simulink model "experiment"  (R2016b)
settings: Solver=VariableStepAuto  StartTime=0.0  StopTime=15  MaxStep=0.05  RelTol=1e-3
model workspace (MAT data in the model file):
  GREEN_TIME = Simulink.Parameter
  GREEN_TIME.Value = 4
  GREEN_TIME.DataType = 'double'
  GREEN_TIME.Dimensions = [1 1]
  MIN_SAFE_DIST = Simulink.Parameter
  MIN_SAFE_DIST.Value = 1
  MIN_SAFE_DIST.DataType = 'double'
  MIN_SAFE_DIST.Dimensions = [1 1]
  PCROSS_TIME = Simulink.Parameter
  PCROSS_TIME.Value = 3
  PCROSS_TIME.DataType = 'double'
  PCROSS_TIME.Dimensions = [1 1]
  V_MIN = Simulink.Parameter
  V_MIN.Value = 0.25
  V_MIN.DataType = 'double'
  V_MIN.Dimensions = [1 1]
  V_TURN = Simulink.Parameter
  V_TURN.Value = 1.2
  V_TURN.DataType = 'double'
  V_TURN.Dimensions = [1 1]
  WORLD_SIZE = Simulink.Parameter
  WORLD_SIZE.Value = 8
  WORLD_SIZE.DataType = 'double'
  WORLD_SIZE.Dimensions = [1 1]
  YELLOW_TIME = Simulink.Parameter
  YELLOW_TIME.Value = 1
  YELLOW_TIME.DataType = 'double'
  YELLOW_TIME.Dimensions = [1 1]
  dt = Simulink.Parameter
  dt.Value = 0.05
  dt.DataType = 'double'
  dt.DocUnits = 'sec'
  dt.Dimensions = [1 1]
values from neighbouring files (symbols this model uses):
  D = ch.find('-isa','Stateflow.Data','-and','Name','D')    [createVehicle.m]    (also in initModelParams.m)
  MIN_SAFE_DIST = 1    [stateflowSim.m]
  V = ch.find('-isa','Stateflow.Data','-and','Name','V')    [createVehicle.m]    (also in initModelParams.m)
  WORLD_SIZE = 8    [offlineSim.m]    (also in stateflowSim.m)
  X = ch.find('-isa','Stateflow.Data','-and','Name','X')    [createVehicle.m]    (also in initModelParams.m)
undefined symbols (not defined in the file or in its folder): Stateflow
libraries: libraries x25
settings Model: Creator=larry  LastModifiedBy=larry
settings SolverCC: ZeroCrossControl=DisableAll  AutoInsertRateTranBlk=on

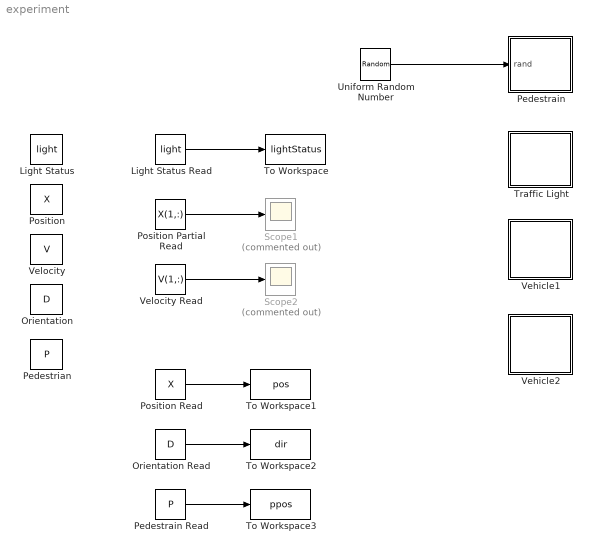
== system experiment ==
  Light Status : DataStoreMemory  DataStoreName=light  ShowAdditionalParam=off  OutDataTypeStr=double  Dimensions=1
  Light Status Read : DataStoreRead  DataStoreName=light
  Orientation : DataStoreMemory  DataStoreName=D  InitialValue=[1 1;0 0]  ShowAdditionalParam=off  OutDataTypeStr=double
  Orientation Read : DataStoreRead  DataStoreName=D
  Pedestrain : Stateflow chart  TreatAsAtomicUnit=on
  Pedestrain Read : DataStoreRead  DataStoreName=P
  Pedestrian : DataStoreMemory  DataStoreName=P  InitialValue=[-1; -1; -1; -1]  ShowAdditionalParam=off  OutDataTypeStr=double
  Position : DataStoreMemory  DataStoreName=X  InitialValue=[-5 -4;-0.5 -0.5]  ShowAdditionalParam=off  OutDataTypeStr=double
  Position Read : DataStoreRead  DataStoreName=X
  Position Partial Read : DataStoreRead  DataStoreName=X  DataStoreElements=X(1,:)
  Scope1 : Scope  Commented=on
  Scope2 : Scope  Commented=on
  To Workspace : ToWorkspace  VariableName=lightStatus  SampleTime=-1
  To Workspace1 : ToWorkspace  VariableName=pos  SampleTime=-1
  To Workspace2 : ToWorkspace  VariableName=dir  SampleTime=-1
  To Workspace3 : ToWorkspace  VariableName=ppos  SampleTime=-1
  Traffic Light : Stateflow chart  TreatAsAtomicUnit=on
  Uniform Random Number : UniformRandomNumber  Minimum=0  Maximum=5  SampleTime=0.05
  Vehicle1 : Stateflow chart  TreatAsAtomicUnit=on
  Vehicle2 : Stateflow chart  TreatAsAtomicUnit=on
  Velocity : DataStoreMemory  DataStoreName=V  InitialValue=[0 0;0 0]  ShowAdditionalParam=off  OutDataTypeStr=double
  Velocity Read : DataStoreRead  DataStoreName=V  DataStoreElements=V(1,:)
  wires:
  Light Status Read/1 -> To Workspace/1
  Position Partial Read/1 -> Scope1/1
  Velocity Read/1 -> Scope2/1
  Position Read/1 -> To Workspace1/1
  Orientation Read/1 -> To Workspace2/1
  Uniform Random Number/1 -> Pedestrain/1(rand)
  Pedestrain Read/1 -> To Workspace3/1

== stateflow chart experiment/Vehicle1 ==
  note: Decision
  note: Perception
  note: Helper
  state GoStraight
    state FreeDriving
    state Follow
      en:
      front = frontCarIndex(this);
      state FollowBehind
    (default) -> GoStraight.FreeDriving [order 2]
    GoStraight.FreeDriving -> GoStraight.Follow : [hasFrontCar(this)]
    GoStraight.Follow -> GoStraight.FreeDriving : [frontCarHasLeft(this)]
    (default) -> GoStraight.Follow [order 1] : [hasFrontCar(this)]
  state Turn
    en:
    completed = false;
    state Right
      en:
      [pf,df] = ...
      prepareRight(this);
      ex:
      inter = resumeFromRight(this, df);
      state Turn
      state TurnStop
      (default) -> Turn.Right.Turn
      Turn.Right.TurnStop -> Turn.Right.Turn : [~hasPedestrian(this)]
      Turn.Right.Turn -> Turn.Right.TurnStop : [hasPedestrian(this)]
    state Left
      en:
      [pf, df] = ...
      prepareLeft(this);
      ex:
      inter = resumeFromLeft(this, df);
      state Turn
      state TurnStop
      (default) -> Turn.Left.Turn
      Turn.Left.TurnStop -> Turn.Left.Turn : [~hasPedestrian(this)]
      Turn.Left.Turn -> Turn.Left.TurnStop : [hasPedestrian(this)]
    (default) -> Right [order 1] : [decision == Decision.Right]
    (default) -> Left [order 2]
  state RoadIntersection
    state Normal
      state FreeDriving
        state AccToHighestRate
        state SlowDownToStop
        state SlowAdjust
        state RushToPass
        (default) -> (junction 88) [order 2]
        (default) -> AccToHighestRate [order 1] : [isGreen(this)]
        AccToHighestRate -> (junction 88) : [isYellow(this)]
        (junction 88) -> (junction 177) [order 2]
        (junction 88) -> RoadIntersection.Normal.FreeDriving.SlowAdjust [order 1] : [isStopped(this)]...
            | {obj = inter;}
        RoadIntersection.Normal.FreeDriving.SlowAdjust -> AccToHighestRate : [isGreen(this)]
        SlowDownToStop -> AccToHighestRate : [isGreen(this)]
        (junction 177) -> SlowDownToStop [order 1] : [isStoppable(this,inter)]...
            | {a_norm = requiredBrake(...
            | this,inter);}
        (junction 177) -> RushToPass [order 2]
      state Follow
        en:
        front = frontCarIndex(this);
        obj = X(:,front);
        du:
        obj = closestObj(this, obj, inter);
        state FollowBehind
        state NonStopFollow
        state SlowAdjust
        (default) -> (junction 164) [order 2]
        (default) -> RoadIntersection.Normal.Follow.FollowBehind [order 1] : [isGreen(this)]
        RoadIntersection.Normal.Follow.FollowBehind -> (junction 164) : [isYellow(this)]
        (junction 164) -> RoadIntersection.Normal.Follow.SlowAdjust [order 1] : [isStoppable(this,obj)]
        (junction 164) -> NonStopFollow [order 2]
        RoadIntersection.Normal.Follow.SlowAdjust -> RoadIntersection.Normal.Follow.FollowBehind : [isGreen(this)]
      (default) -> RoadIntersection.Normal.FreeDriving [order 2]
      (default) -> RoadIntersection.Normal.Follow [order 1] : [hasFrontCar(this)]
      RoadIntersection.Normal.FreeDriving -> RoadIntersection.Normal.Follow : [hasFrontCar(this)]
      RoadIntersection.Normal.Follow -> RoadIntersection.Normal.FreeDriving : [frontCarHasLeft(this)]
    state Pedestrian
      state EmergenceStop
    (default) -> Normal [order 2]
    Normal -> Pedestrian : [hasPedestrian(this)]
    Pedestrian -> Normal : [~hasPedestrian(this)]
    (default) -> Pedestrian [order 1] : [hasPedestrian(this)]
  (default) -> GoStraight
  Turn -> GoStraight : [completed]
  (junction 195) -> Turn [order 2]
  (junction 195) -> GoStraight [order 1] : [decision == Decision.Straight]
  RoadIntersection -> (junction 195) : [passStopLine(this)]
  GoStraight -> RoadIntersection : [isCloseTo(this,inter)]
  data: v_target function_input; a_norm function_input; this function_input; a_max function_input; this function_input; front function_input; this function_input; completed function_output; d2 function_input; p2 function_input; this function_input; p2 function_input; this function_input; completed function_output; d2 function_input; p2 function_input; this function_input; p2 function_input; self function_input; res function_output; self function_input; obj1 function_input; res function_output; obj2 function_input; self function_input; pos function_input; res function_output; self function_input; res function_output; self function_input; idx function_output; self function_input uint8 size=1; d function_input; newInnter function_output; self function_input; res function_output; pos function_input; self function_input; pos function_input; res function_output; self function_input uint8 size=1; d function_input; newInter function_output; self function_input; res function_output; self function_input uint8 size=1; p function_output; d function_output; self function_input uint8 size=1; p function_output; d function_output; self function_input; res function_output; self function_input; res function_output; self function_input; res function_output; v_target function_input; a_norm function_input; this function_input; a_norm function_input; this function_input; this function_input; a_norm function_input; obj function_input; v_target function_input; a_norm function_input; this function_input; a_max function_input; this function_input; front function_input; a_max function_input; this function_input; front function_input; this function_input; a_norm function_input; obj function_input; a_norm function_input; this function_input; self function_input uint8 size=1; res function_output boolean size=1; dt parameter double size=1 =0.05; this local uint8 =uint8(1); V data_store_memory; X data_store_memory size=[1 2]; D data_store_memory; A_MAX local double =2.5; V_MAX local double =2.5; light data_store_memory; inter local double size=[2 1] =[-1; -0.5]; MIN_SAFE_DIST parameter; a_norm local double size=1 =0; WORLD_SIZE parameter; front local uint8 size=1; obj local double size=[2 1]; V_MIN parameter; decision local Enum: Decision size=1 =Decision.Right; completed local boolean size=1 =false; P data_store_memory; df local double size=[2 1]; pf local double size=[2 1]
  function res = hasPedestrian(self):
    | function res = hasPedestrian(self)
    | 
    | if ~any(P ~= -1)
    |     res = false;
    |     return;
    | end
    | 
    | FARAWAY = 100;
    | 
    | pi = [-1 1 1 -1; -1 -1 1 1];
    | dp = [2 0 -2 0; 0 2 0 -2];
    | 
    | dx_norm = ones(4, 1) * FARAWAY;
    | x = X(:,self);
    | d = D(:,self);
    | 
    | for k=1:length(P)
    |     if P(k) ~= -1
    |         p = pi(:,k) + dp(:,k) * P(k); 
    |         dx = p - x;
    |         check = dot(dx, d);
    |         if check > 0
    |             dx_norm(k) = norm(dx);
    |             theta = acos(check/dx_norm(k));
    |             if rad2deg(theta) > 10
    |                 dx_norm(k) = FARAWAY;
    |             end
    |         end
    |     end
    | end
    | 
    | res = any(dx_norm <= 1 * MIN_SAFE_DIST);
  function res = closestObj(self, obj1, obj2):
    | function res = closestObj(self, obj1, obj2)
    | 
    | if isequal(obj1, obj2)
    |     res = obj1;
    |     return;
    | end
    | 
    | RANGE = 2*WORLD_SIZE;
    | 
    | x = X(:,self);
    | d = D(:,self);
    | 
    | dX = zeros(2, 1);
    | dX(1) = mod(dot(obj1 - x, d) + RANGE, RANGE);
    | dX(2) = mod(dot(obj2 - x, d) + RANGE, RANGE);
    | 
    | [~, index] = min(dX);
    | if index == 1
    |     res = obj1;
    | else
    |     res = obj2;
    | end
  function res = isStoppable(self,pos):
    | function res = isStoppable(self,pos)
    | 
    | x = X(:,self);
    | v = V(:,self);
    | d = D(:,self);
    | 
    | range = 2 * WORLD_SIZE;
    | diff = mod((dot(pos - x, d)+range), range) ;
    | dist = diff - MIN_SAFE_DIST;
    | 
    | v_norm = norm(v);
    | brake_dist = v_norm*v_norm/2.0/A_MAX;
    | res = (brake_dist <= dist);
  function res = passStopLine(self):
    | function res = passStopLine(self)
    | 
    | x = X(:,self);
    | d = D(:,self);
    | 
    | dx_norm = dot(inter - x, d);
    | res = (dx_norm <= 0);
  function idx = frontCarIndex(self):
    | function idx = frontCarIndex(self)
    | 
    | FARAWAY = 100;
    | RANGE = 2*WORLD_SIZE;
    | 
    | dx = zeros(size(X, 2), 1);
    | x = X(:,self);
    | v = V(:,self);
    | d = D(:,self);
    | 
    | for k=1:length(dx)
    |     dx(k) = dot(X(:,k) - x, d);
    |     dx(k) = mod((dx(k)+RANGE), RANGE);
    | end
    | 
    | % set zero dX to a large enough value
    | dx(dx == 0) = FARAWAY;
    | [~, idx] = min(dx);
    | idx = uint8(idx);
  function newInnter = resumeFromRight(self, d):
    | function newInnter = resumeFromRight(self, d)
    | 
    | x = X(:,self);
    | 
    | if isequal(d, [0; -1])
    |     x = [-0.5; -1];
    |     newInnter = [-0.5; 1];
    | elseif isequal(d, [0; 1])
    |     x = [0.5; 1];
    |     newInnter = [-0.5; -1];
    | elseif isequal(d, [1; 0])
    |     x = [1; -0.5];
    |     newInnter = [-1; -0.5];
    | elseif isequal(d, [-1; 0])
    |     x = [-1; 0.5];
    |     newInnter = [1; 0.5];
    | else
    |     error('Unknown orientation');
    | end
    | 
    | v = V(:,self);
    | 
    | X(:,self) = x;
    | V(:,self) = d * norm(v);
    | D(:,self) = d;
  function res = isCloseTo(self,pos):
    | function res = isCloseTo(self,pos)
    | 
    | x = X(:,self);
    | d = D(:,self);
    | 
    | dist = dot(pos-x, d);
    | res = ((dist > 0) && (dist <= 2.5*MIN_SAFE_DIST));
  function res = requiredBrake(self,pos):
    | function res = requiredBrake(self,pos)
    | 
    | x = X(:,self);
    | v = V(:,self);
    | d = D(:,self);
    | 
    | % add safe distance
    | range = 2 * WORLD_SIZE;
    | diff = mod((dot(pos - x, d)+range),range);
    | dist = diff - MIN_SAFE_DIST;
    | assert(dist >= 0);
    | 
    | vnorm = norm(v);
    | res = vnorm*vnorm/2/dist;
  function newInter = resumeFromLeft(self, d):
    | function newInter = resumeFromLeft(self, d)
    | 
    | x = X(:,self);
    | v = V(:,self);
    | 
    | if isequal(d, [1; 0])
    |     x = [1; -0.5];
    |     newInter = [-1; -0.5];
    | elseif isequal(d, [-1; 0])
    |     x = [-1; 0.5];
    |     newInter = [1; 0.5];
    | elseif isequal(d, [0; 1])
    |     x = [0.5; 1];
    |     newInter = [0.5; -1];
    | elseif isequal(d, [0; -1])
    |     x = [-0.5; -1];
    |     newInter = [-0.5; 1];
    | else
    |     error('Unknown orientation');
    | end
    | 
    | X(:,self) = x;
    | V(:,self) = d * norm(v);
    | D(:,self) = d;
  function res = isGreen(self):
    | function res = isGreen(self)
    | 
    | d = D(:,self);
    | 
    | % compute the corresponding traffic light
    | horizon = (abs(d(1)) ~= 0);
    | vertical = (abs(d(2)) ~= 0);
    | 
    | res = false;
    | if uint8(light) == 3 && horizon
    |     % horizontal: green, vertical: red
    |     res = true;
    | elseif uint8(light) == 1 && vertical
    |     % horizontal: red, vertical: green
    |     res = true;
    | end
  function [p, d] = prepareRight(self):
    | function [p, d] = prepareRight(self)
    | 
    | d0 = D(:,self);
    | p = [0; 0];
    | d = [0; 0];
    | 
    | if isequal(d0, [1; 0])
    |     p = [-0.5; -1];
    |     d = [0; -1];
    | elseif isequal(d0, [-1; 0])
    |     p = [0.5; 1];
    |     d = [0; 1];
    | elseif isequal(d0, [0; 1])
    |     p = [1; -0.5];
    |     d = [1; 0];
    | elseif isequal(d0, [0; -1])
    |     p = [-1; 0.5];
    |     d = [-1; 0];
    | else
    |     error('Unknown orientation');
    | end
  function [p, d] = prepareLeft(self):
    | function [p, d] = prepareLeft(self)
    | 
    | d0 = D(:,self);
    | p = [0; 0];
    | d = [0; 0];
    | 
    | if isequal(d0, [1; 0])
    |     p = [0.5; 1];
    |     d = [0; 1];
    | elseif isequal(d0, [-1; 0])
    |     p = [-0.5; -1];
    |     d = [0; -1];
    | elseif isequal(d0, [0; 1])
    |     p = [-1; 0.5];
    |     d = [-1; 0];
    | elseif isequal(d0, [0; -1])
    |     p = [1; -0.5];
    |     d = [1; 0];
    | else
    |     error('Unknown orientation');
    | end
  function res = isYellow(self):
    | function res = isYellow(self)
    | 
    | d = D(:,self);
    | 
    | % compute the corresponding traffic light
    | horizon = (abs(d(1)) ~= 0);
    | vertical = (abs(d(2)) ~= 0);
    | 
    | res = false;
    | if uint8(light) == 4 && horizon
    |     % horizontal: yellow, vertical: red
    |     res = true;
    | elseif uint8(light) == 2 && vertical
    |     % horizontal: red, vertical: yellow
    |     res = true;
    | end
  function res = hasFrontCar(self):
    | function res = hasFrontCar(self)
    | 
    | % constants
    | THRES = 2 * MIN_SAFE_DIST;
    | FARAWAY = 100;
    | RANGE = 2 * WORLD_SIZE;
    | 
    | res = false;
    | 
    | % row of X: coordinate, col of X: num of cars
    | num = size(X, 2);
    | if num == 1
    |     return;
    | end
    | 
    | dx = zeros(num, 1);
    | x = X(:,self);
    | d = D(:,self);
    | car_size = [0.3; 0.4];
    | 
    | for k=1:length(dx)
    |     
    |     % compute difference
    |     xdelta = X(:,k) - x;
    |     
    |     % parallel and vertical distance
    |     delta_p = dot(xdelta, d);
    |     delta_v = norm(xdelta - (d * delta_p));
    |     
    |     % vertical distance is larger than car width
    |     if delta_v < car_size(1)
    |         dx(k) = delta_p;
    |     else
    |         dx(k) = FARAWAY;
    |     end
    |     
    |     % a rounded world
    |     dx(k) = mod((dx(k)+RANGE), RANGE);
    | end
    | 
    | % set zero dX to a large enough value
    | dx(dx == 0) = FARAWAY;
    | closest = min(dx);
    | res = closest <= THRES;
  function res = frontCarHasLeft(self):
    | function res = frontCarHasLeft(self)
    | 
    | % Constants 
    | THRES = 2.5 * MIN_SAFE_DIST;
    | FARAWAY = 100;
    | RANGE = 2 * WORLD_SIZE;
    | 
    | % if only one car in the environment return directly
    | res = true;
    | num = size(X, 1);
    | if num == 1
    |     return;
    | end
    | 
    | % get the closet car index and its distance
    | dx = zeros(num, 1);
    | x = X(:,self);
    | d = D(:,self);
    | car_size = [0.3; 0.4];
    | 
    | for k=1:length(dx)
    |     
    |     xdelta = X(:,k) - x;
    |     xdelta_p = dot(xdelta, d);                  % parallel component
    |     xdelta_v = norm(xdelta - (d * xdelta_p));   % vertical component
    |     
    |     % when the vertical component is larger than the car width
    |     if xdelta_v < car_size(1)
    |         dx(k) = xdelta_p;
    |     else
    |         dx(k) = FARAWAY;
    |     end
    |     
    |     % since we are in the round world, normalize the distance if the 
    |     % front car is behind us 
    |     % a rounded world
    |     dx(k) = mod((dx(k)+RANGE), RANGE);
    | end
    | 
    | % set the zero dx to a large enough value for convenience
    | dx(dx == 0) = FARAWAY;
    | closest = min(dx);
    | res = closest > THRES;
  function res = isStopped(self):
    | function res = isStopped(self)
    | 
    | v = V(:,self);
    | d = D(:,self);
    | res = (dot(v, d) <= 0)||(norm(v) < V_MIN);

== stateflow chart experiment/Vehicle2 ==
  state Turn
    en:
    theta_in = 0;
    completed = false;
    state TurnLeft
    state TurnRight
    (default) -> TurnLeft [order 2]
    (default) -> TurnRight [order 1] : [decision == Decision.Right]
  state GoStraight
    state FreeDriving
    state Follow
      en:
      front = frontCarIndex(this);
      state FollowBehind
    (default) -> GoStraight.FreeDriving [order 2]
    GoStraight.FreeDriving -> GoStraight.Follow : [hasFrontCar(this)]
    GoStraight.Follow -> GoStraight.FreeDriving : [frontCarHasLeft(this)]
    (default) -> GoStraight.Follow [order 1] : [hasFrontCar(this)]
  state RoadIntersection
    state FreeDriving
      state AccToHighestRate
      state SlowDownToStop
      state SlowAdjust
      state RushToPass
      (default) -> (junction 88) [order 2]
      (default) -> AccToHighestRate [order 1] : [isGreen(this)]
      AccToHighestRate -> (junction 88) : [isYellow(this)]
      (junction 88) -> (junction 177) [order 2]
      (junction 88) -> RoadIntersection.FreeDriving.SlowAdjust [order 1] : [isStopped(this)]...
          | {obj = inter;}
      RoadIntersection.FreeDriving.SlowAdjust -> AccToHighestRate : [isGreen(this)]
      SlowDownToStop -> AccToHighestRate : [isGreen(this)]
      (junction 177) -> SlowDownToStop [order 1] : [isStoppable(this,inter)]...
          | {a_norm = requiredBrake(...
          | this,inter);}
      (junction 177) -> RushToPass [order 2]
    state Follow
      en:
      front = frontCarIndex(this);
      obj = X(:,front);
      du:
      obj = closestObj(this, obj, inter);
      state FollowBehind
      state NonStopFollow
      state SlowAdjust
      (default) -> (junction 164) [order 2]
      (default) -> RoadIntersection.Follow.FollowBehind [order 1] : [isGreen(this)]
      RoadIntersection.Follow.FollowBehind -> (junction 164) : [isYellow(this)]
      (junction 164) -> RoadIntersection.Follow.SlowAdjust [order 1] : [isStoppable(this,obj)]
      (junction 164) -> NonStopFollow [order 2]
      RoadIntersection.Follow.SlowAdjust -> RoadIntersection.Follow.FollowBehind : [isGreen(this)]
    (default) -> RoadIntersection.FreeDriving [order 2]
    (default) -> RoadIntersection.Follow [order 1] : [hasFrontCar(this)]
    RoadIntersection.FreeDriving -> RoadIntersection.Follow : [hasFrontCar(this)]
    RoadIntersection.Follow -> RoadIntersection.FreeDriving : [frontCarHasLeft(this)]
  (default) -> GoStraight
  Turn -> GoStraight : [completed]
  (junction 195) -> Turn [order 2]
  (junction 195) -> GoStraight [order 1] : [decision == Decision.Straight]
  RoadIntersection -> (junction 195) : [passStopLine(this)]
  GoStraight -> RoadIntersection : [isCloseTo(this,inter)]
  data: newInter function_output; this function_input; completed function_output; newInter function_output; this function_input; completed function_output; theta_in function_input; theta function_output; v_target function_input; a_norm function_input; this function_input; a_max function_input; this function_input; front function_input; self function_input; res function_output; self function_input; res function_output; self function_input; res function_output; pos function_input; self function_input; res function_output; self function_input; res function_output; self function_input; res function_output; self function_input; res function_output; v_target function_input; a_norm function_input; this function_input; a_norm function_input; this function_input; this function_input; a_norm function_input; obj function_input; v_target function_input; a_norm function_input; this function_input; a_max function_input; this function_input; front function_input; a_max function_input; this function_input; front function_input; this function_input; a_norm function_input; obj function_input; self function_input; obj1 function_input; res function_output; obj2 function_input; self function_input; idx function_output; self function_input; pos function_input; res function_output; self function_input; pos function_input; res function_output; self function_input uint8 size=1; res function_output boolean size=1; dt parameter double size=1 =0.05; this local uint8 =uint8(2); V data_store_memory; X data_store_memory size=[1 2]; D data_store_memory; A_MAX local double =2.5; V_MAX local double =2.5; light data_store_memory; inter local double size=[2 1] =[-1; -0.5]; MIN_SAFE_DIST parameter; a_norm local double size=1 =0; WORLD_SIZE parameter; front local uint8 size=1; obj local double size=[2 1]; V_MIN parameter; decision local Enum: Decision size=1 =Decision.Straight; completed local boolean size=1 =false; theta_in local double size=1 =0; theta_out local double size=1 =0
  function res = hasPedestrian(self):
    | function res = hasPedestrian(self)
    | 
    | FARAWAY = 100;
    | 
    | pi = [-1 1 1 -1; -1 -1 1 1];
    | dp = [2 0 -2 0; 0 2 0 -2];
    | 
    | dx_norm = ones(4, 1) * FARAWAY;
    | x = X(:,self);
    | d = D(:,self);
    | 
    | for k=1:length(P)
    |     if P(k) ~= -1
    |         p = pi(:,k) + dp * P(k); 
    |         dx = p - x;
    |         if dot(dx, d) > 0
    |             dx_norm(k) = norm(dx);
    |         end
    |     end
    | end
    | res = ~isempty(dx <= MIN_SAFE_DIST);
  function res = passStopLine(self):
    | function res = passStopLine(self)
    | 
    | x = X(:,self);
    | d = D(:,self);
    | 
    | dx_norm = dot(inter - x, d);
    | res = (dx_norm <= 0);
  function res = isCloseTo(self,pos):
    | function res = isCloseTo(self,pos)
    | 
    | x = X(:,self);
    | d = D(:,self);
    | 
    | dist = dot(pos-x, d);
    | res = ((dist > 0) && (dist <= 2.5*MIN_SAFE_DIST));
  function res = isGreen(self):
    | function res = isGreen(self)
    | 
    | d = D(:,self);
    | 
    | % compute the corresponding traffic light
    | horizon = (abs(d(1)) ~= 0);
    | vertical = (abs(d(2)) ~= 0);
    | 
    | res = false;
    | if uint8(light) == 3 && horizon
    |     % horizontal: green, vertical: red
    |     res = true;
    | elseif uint8(light) == 1 && vertical
    |     % horizontal: red, vertical: green
    |     res = true;
    | end
  function res = isYellow(self):
    | function res = isYellow(self)
    | 
    | d = D(:,self);
    | 
    | % compute the corresponding traffic light
    | horizon = (abs(d(1)) ~= 0);
    | vertical = (abs(d(2)) ~= 0);
    | 
    | res = false;
    | if uint8(light) == 4 && horizon
    |     % horizontal: yellow, vertical: red
    |     res = true;
    | elseif uint8(light) == 2 && vertical
    |     % horizontal: red, vertical: yellow
    |     res = true;
    | end
  function res = hasFrontCar(self):
    | function res = hasFrontCar(self)
    | 
    | % constants
    | THRES = 2 * MIN_SAFE_DIST;
    | FARAWAY = 100;
    | RANGE = 2 * WORLD_SIZE;
    | 
    | res = false;
    | 
    | % row of X: coordinate, col of X: num of cars
    | num = size(X, 2);
    | if num == 1
    |     return;
    | end
    | 
    | dx = zeros(num, 1);
    | x = X(:,self);
    | d = D(:,self);
    | car_size = [0.3; 0.4];
    | 
    | for k=1:length(dx)
    |     
    |     % compute difference
    |     xdelta = X(:,k) - x;
    |     
    |     % parallel and vertical distance
    |     delta_p = dot(xdelta, d);
    |     delta_v = norm(xdelta - (d * delta_p));
    |     
    |     % vertical distance is larger than car width
    |     if delta_v < car_size(1)
    |         dx(k) = delta_p;
    |     else
    |         dx(k) = FARAWAY;
    |     end
    |     
    |     % a rounded world
    |     dx(k) = mod((dx(k)+RANGE), RANGE);
    | end
    | 
    | % set zero dX to a large enough value
    | dx(dx == 0) = FARAWAY;
    | closest = min(dx);
    | res = closest <= THRES;
  function res = frontCarHasLeft(self):
    | function res = frontCarHasLeft(self)
    | 
    | % Constants 
    | THRES = 2.5 * MIN_SAFE_DIST;
    | FARAWAY = 100;
    | RANGE = 2 * WORLD_SIZE;
    | 
    | % if only one car in the environment return directly
    | res = true;
    | num = size(X, 1);
    | if num == 1
    |     return;
    | end
    | 
    | % get the closet car index and its distance
    | dx = zeros(num, 1);
    | x = X(:,self);
    | d = D(:,self);
    | car_size = [0.3; 0.4];
    | 
    | for k=1:length(dx)
    |     
    |     xdelta = X(:,k) - x;
    |     xdelta_p = dot(xdelta, d);                  % parallel component
    |     xdelta_v = norm(xdelta - (d * xdelta_p));   % vertical component
    |     
    |     % when the vertical component is larger than the car width
    |     if xdelta_v < car_size(1)
    |         dx(k) = xdelta_p;
    |     else
    |         dx(k) = FARAWAY;
    |     end
    |     
    |     % since we are in the round world, normalize the distance if the 
    |     % front car is behind us 
    |     % a rounded world
    |     dx(k) = mod((dx(k)+RANGE), RANGE);
    | end
    | 
    | % set the zero dx to a large enough value for convenience
    | dx(dx == 0) = FARAWAY;
    | closest = min(dx);
    | res = closest > THRES;
  function res = closestObj(self, obj1, obj2):
    | function res = closestObj(self, obj1, obj2)
    | 
    | if isequal(obj1, obj2)
    |     res = obj1;
    |     return;
    | end
    | 
    | RANGE = 2*WORLD_SIZE;
    | 
    | x = X(:,self);
    | d = D(:,self);
    | 
    | dX = zeros(2, 1);
    | dX(1) = mod(dot(obj1 - x, d) + RANGE, RANGE);
    | dX(2) = mod(dot(obj2 - x, d) + RANGE, RANGE);
    | 
    | [~, index] = min(dX);
    | if index == 1
    |     res = obj1;
    | else
    |     res = obj2;
    | end
  function idx = frontCarIndex(self):
    | function idx = frontCarIndex(self)
    | 
    | FARAWAY = 100;
    | RANGE = 2*WORLD_SIZE;
    | 
    | dx = zeros(size(X, 2), 1);
    | x = X(:,self);
    | v = V(:,self);
    | d = D(:,self);
    | 
    | for k=1:length(dx)
    |     dx(k) = dot(X(:,k) - x, d);
    |     dx(k) = mod((dx(k)+RANGE), RANGE);
    | end
    | 
    | % set zero dX to a large enough value
    | dx(dx == 0) = FARAWAY;
    | [~, idx] = min(dx);
    | idx = uint8(idx);
  function res = isStoppable(self,pos):
    | function res = isStoppable(self,pos)
    | 
    | x = X(:,self);
    | v = V(:,self);
    | d = D(:,self);
    | 
    | range = 2 * WORLD_SIZE;
    | diff = mod((dot(pos - x, d)+range), range) ;
    | dist = diff - MIN_SAFE_DIST;
    | 
    | v_norm = norm(v);
    | brake_dist = v_norm*v_norm/2.0/A_MAX;
    | res = (brake_dist <= dist);
  function res = requiredBrake(self,pos):
    | function res = requiredBrake(self,pos)
    | 
    | x = X(:,self);
    | v = V(:,self);
    | d = D(:,self);
    | 
    | % add safe distance
    | range = 2 * WORLD_SIZE;
    | diff = mod((dot(pos - x, d)+range),range);
    | dist = diff - MIN_SAFE_DIST;
    | assert(dist >= 0);
    | 
    | vnorm = norm(v);
    | res = vnorm*vnorm/2/dist;
  function res = isStopped(self):
    | function res = isStopped(self)
    | 
    | v = V(:,self);
    | d = D(:,self);
    | res = (dot(v, d) <= 0)||(norm(v) < V_MIN);

== stateflow chart experiment/Traffic Light ==
  state Y_R
    en:
    light = 4;
  state R_G
    en:
    light = 1;
    state Pass
    state NotPass
    (default) -> R_G.Pass
    R_G.Pass -> R_G.NotPass : after(G_TIME-CROSS_TIME,sec)
  state G_R
    en:
    light = 3;
    state Pass
    state NotPass
    (default) -> G_R.Pass
    G_R.Pass -> G_R.NotPass : after(G_TIME-CROSS_TIME,sec)
  state R_Y
    en:
    light = 2;
  Y_R -> R_G : after(Y_TIME, sec)
  G_R -> Y_R : after(G_TIME, sec)
  (default) -> R_G
  R_G -> R_Y : after(G_TIME, sec)
  R_Y -> G_R : after(Y_TIME, sec)
  data: light data_store_memory; CROSS_TIME constant double =3; G_TIME constant double =4; Y_TIME constant double =1

== stateflow chart experiment/Pedestrain ==
  state P_LeftBottom
    state Walking
      en:
      P(this) = 0;
      du:
      P(this) = ...
      temporalCount(sec)/PCROSS_TIME;
      ex:
      P(this) = 1;
    state Finish
      en:
      P(this) = -1;
    state Wait
    Walking -> Finish : after(PCROSS_TIME, sec)
    Wait -> Walking : [light == 3]
    Finish -> Wait : [uint8(rand) == this]
    (default) -> Finish
  (default) -> P_LeftBottom
  data: this local uint8 size=1 =uint8(1); light data_store_memory; PCROSS_TIME parameter; P data_store_memory; rand input
